simulink model "Adeline"  (Simulink 7.5)
settings: Solver=ode45  StartTime=0.0  StopTime=10.0  RelTol=1e-3
settings Model: Creator=My Laptop  LastModifiedBy=My Laptop

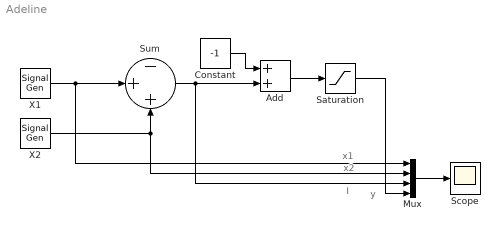
== system Adeline ==
  note: y
  note: I
  note: x1
  note: x2
  Add : Sum  OutDataType=fixdt(1, 16)  OutScaling=2^-10
  Constant : Constant  Value=-1  OutDataType=fixdt(1, 16)  OutScaling=2^0
  Mux : Mux
  Saturation : Saturate  UpperLimit=1  LowerLimit=-1  ZeroCross=off  OutDataType=fixdt(1, 16)  OutScaling=2^0
  Scope : Scope
      settings: YMin=-3  YMax=3
  Sum : Sum  Inputs=-++  OutDataType=fixdt(1, 16)  OutScaling=2^0
  X1 : SignalGenerator  WaveForm=square  Frequency=.4
  X2 : SignalGenerator  WaveForm=square  Frequency=.2
  wires:
  Mux/1 -> Scope/1
  Sum/1 -> Mux/3, Add/2
  X2/1 -> Sum/3, Mux/2
  X1/1 -> Mux/1, Sum/2
  Saturation/1 -> Mux/4
  Constant/1 -> Add/1
  Add/1 -> Saturation/1
